simulink model "tp_simulink"  (R2015a)
settings: Solver=ode45  StartTime=0.0  StopTime=5  RelTol=1e-3
libraries: dspvision x4, dspadpt3 x4, dspindex x1
settings Model: Creator=admin  LastModifiedBy=admin

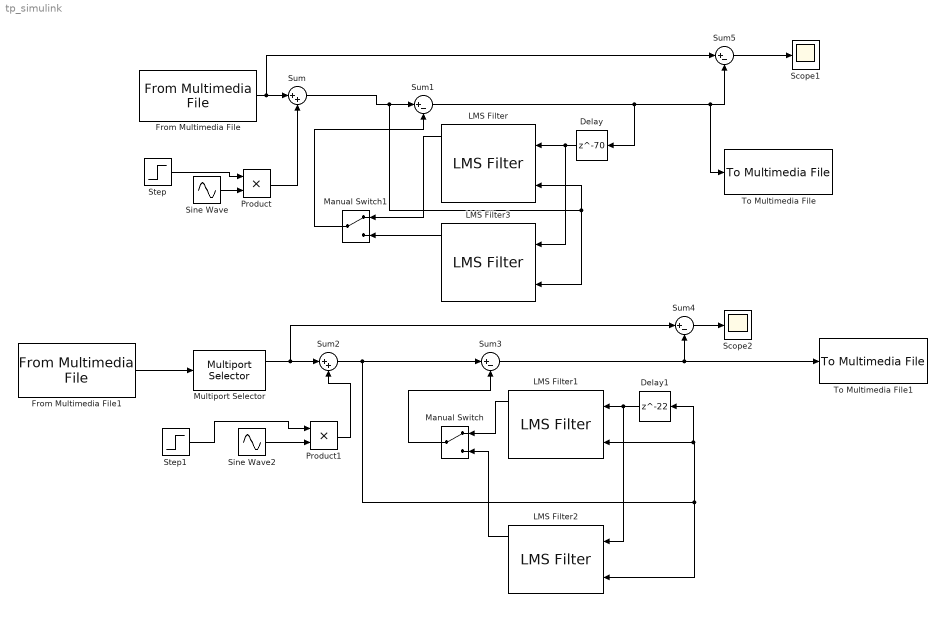
== system tp_simulink ==
  Delay : Delay  DelayLength=70
  Delay1 : Delay  DelayLength=22  InitialCondition=0
  From Multimedia File : dspvision/From Multimedia File  inputFilename=speech_dft.mp3  loop=on  numPlays=1  outputStreams=Audio only  videoDataType=single  audioDataType=double  inheritSampleTime=off  userDefinedSampleTime=0.00004535147  noAudioOutput=off  isIntensityVideo=off  fourcc=RGB  colorVideoFormat=Separate color signals  outputEOF=off  dataOrg=Column-major  audioFrameSize=1  computeAudioFrameSize=off  outSamplingMode=Sample based
  From Multimedia File1 : dspvision/From Multimedia File  inputFilename=C:\Users\admin\Dropbox\PSII\TpFinal\Alvaro\audio\audio001.mp3  loop=on  numPlays=inf  outputStreams=Audio only  videoDataType=single  audioDataType=double  inheritSampleTime=on  userDefinedSampleTime=1/44100  noAudioOutput=off  isIntensityVideo=off  fourcc=RGB  colorVideoFormat=Separate color signals  outputEOF=off  dataOrg=Column-major  audioFrameSize=1  computeAudioFrameSize=off  outSamplingMode=Sample based
  LMS Filter : dspadpt3/LMS Filter  Algo=Normalized LMS  L=400  stepflag=Dialog  mu=0.03  leakage=1.0  ic=0  Adapt=off  resetflag=None  weights=on  secondCoeffMode=User-defined  secondCoeffWordLength=2  secondCoeffFracLength=15  accum2Mode=User-defined  accum2FracLength=20  prodOutput2Mode=User-defined  prodOutput2FracLength=20  prodOutput3Mode=User-defined  prodOutput3FracLength=20  prodOutput4Mode=User-defined  prodOutput4FracLength=20  quotientMode=User-defined  quotientFracLength=20  roundingMode=Floor  overflowMode=off  addnparflag=off
  LMS Filter1 : dspadpt3/LMS Filter  Algo=LMS  L=400  stepflag=Dialog  mu=0.005  leakage=1.0  ic=0  Adapt=off  resetflag=None  weights=on  secondCoeffMode=User-defined  secondCoeffWordLength=2  secondCoeffFracLength=15  accum2Mode=User-defined  accum2FracLength=20  prodOutput2Mode=User-defined  prodOutput2FracLength=20  prodOutput3Mode=User-defined  prodOutput3FracLength=20  prodOutput4Mode=User-defined  prodOutput4FracLength=20  quotientMode=User-defined  quotientFracLength=20  roundingMode=Floor  overflowMode=off  addnparflag=off
  LMS Filter2 : dspadpt3/LMS Filter  Algo=Normalized LMS  L=400  stepflag=Dialog  mu=0.02  leakage=1.0  ic=0  Adapt=off  resetflag=None  weights=on  secondCoeffMode=User-defined  secondCoeffWordLength=2  secondCoeffFracLength=15  accum2Mode=User-defined  accum2FracLength=20  prodOutput2Mode=User-defined  prodOutput2FracLength=20  prodOutput3Mode=User-defined  prodOutput3FracLength=20  prodOutput4Mode=User-defined  prodOutput4FracLength=20  quotientMode=User-defined  quotientFracLength=20  roundingMode=Floor  overflowMode=off  addnparflag=off
  LMS Filter3 : dspadpt3/LMS Filter  Algo=LMS  L=400  stepflag=Dialog  mu=0.01  leakage=1.0  ic=0  Adapt=off  resetflag=None  weights=on  secondCoeffMode=User-defined  secondCoeffWordLength=2  secondCoeffFracLength=15  accum2Mode=User-defined  accum2FracLength=20  prodOutput2Mode=User-defined  prodOutput2FracLength=20  prodOutput3Mode=User-defined  prodOutput3FracLength=20  prodOutput4Mode=User-defined  prodOutput4FracLength=20  quotientMode=User-defined  quotientFracLength=20  roundingMode=Floor  overflowMode=off  addnparflag=off
  Manual Switch : ManualSwitch
  Manual Switch1 : ManualSwitch
  Multiport Selector : dspindex/Multiport Selector  rowsOrCols=Columns  idxCellArray={1,2}  idxErrMode=Clip Index
  Product : Product
  Product1 : Product
  Scope1 : Scope
      settings: YMin=-1.12631  YMax=1.074
  Scope2 : Scope
      settings: YMin=-1.12631  YMax=1.074
  Sine Wave : Sin  Frequency=2*pi*100  SampleTime=0.00004535147
  Sine Wave2 : Sin  Frequency=2*pi*50  SampleTime=1/44100
  Step : Step  Time=2  SampleTime=0.00004535147
  Step1 : Step  Time=2  SampleTime=1/44100
  Sum : Sum  Inputs=|++
  Sum{1,3..5} (4 alike) : Sum  Inputs=|+-
  Sum2 : Sum  Inputs=|++
  To Multimedia File : dspvision/To Multimedia File  outputFilename=C:\Users\admin\Dropbox\PSII\TpFinal\Alvaro\audio\fbnc_no_loop.wav  streamSelection=Audio only  videoCompressor=None (uncompressed)  audioCompressor=None (uncompressed)  imagePorts=Separate color signals  fileType=WAV  audioDatatype=16-bit integer  fourcc=RGB  videoQuality=75  mj2000CompFactor=10
  To Multimedia File1 : dspvision/To Multimedia File  outputFilename=C:\Users\admin\Dropbox\PSII\TpFinal\Alvaro\audio\apnc_no_loop.wav  streamSelection=Audio only  videoCompressor=None (uncompressed)  audioCompressor=None (uncompressed)  imagePorts=Separate color signals  fileType=WAV  audioDatatype=16-bit integer  fourcc=RGB  videoQuality=75  mj2000CompFactor=10
  wires:
  From Multimedia File/1 -> Sum5/1, Sum/1
  Sine Wave/1 -> Product/2
  Step/1 -> Product/1
  Product/1 -> Sum/2
  Delay/1 -> LMS Filter3/1, LMS Filter/1
  Sum1/1 -> Delay/1, To Multimedia File/1, Sum5/2
  LMS Filter/1 -> Manual Switch1/1
  Sum/1 -> LMS Filter3/2, LMS Filter/2, Sum1/1
  Delay1/1 -> LMS Filter2/1, LMS Filter1/1
  From Multimedia File1/1 -> Multiport Selector/1
  Manual Switch/1 -> Sum3/2
  LMS Filter1/1 -> Manual Switch/1
  LMS Filter2/1 -> Manual Switch/2
  Sum2/1 -> Delay1/1, LMS Filter1/2, LMS Filter2/2, Sum3/1
  LMS Filter3/1 -> Manual Switch1/2
  Manual Switch1/1 -> Sum1/2
  Sum4/1 -> Scope2/1
  Sum3/1 -> Sum4/2, To Multimedia File1/1
  Multiport Selector/1 -> Sum4/1, Sum2/1
  Sum5/1 -> Scope1/1
  Step1/1 -> Product1/1
  Sine Wave2/1 -> Product1/2
  Product1/1 -> Sum2/2
